simulink model "UUV_ss_reg"  (Simulink 8.0)
settings: Solver=ode45  StartTime=0.0  StopTime=10  RelTol=1e-3
values from neighbouring files (symbols this model uses):
  P =     [matlab.mat]
undefined symbols (not defined in the file or in its folder): controller, drawUUV
settings Model: Creator=beard  LastModifiedBy=tmclain
settings DataIOCC: SignalLoggingSaveFormat=ModelDataLogs
settings OptimizationCC: InitFltsAndDblsToZero=on
settings DebuggingCC: FcnCallInpInsideContextMsg=EnableAllAsWarning  StrictBusMsg=Warning
settings GRTTargetCC: CombineOutputUpdateFcns=off  GRTInterface=on

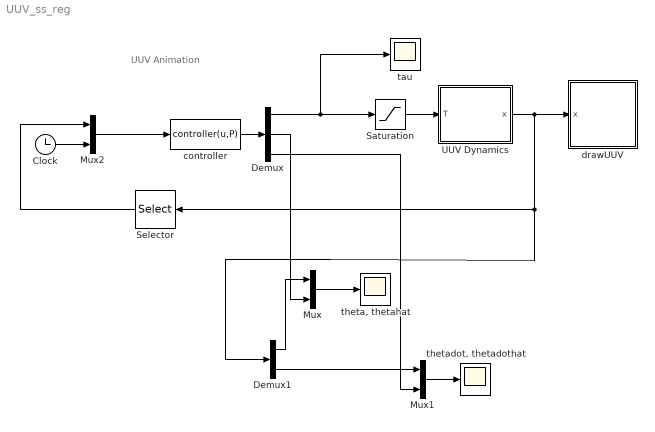
== system UUV_ss_reg ==
  note: UUV Animation
  Clock : Clock
  Demux : Demux  Outputs=3
  Demux1 : Demux  Outputs=2
  Mux : Mux  Inputs=2
  Mux1 : Mux  Inputs=2
  Mux2 : Mux  Inputs=2
  Saturation : Saturate  UpperLimit=250  LowerLimit=-250
  Selector : Selector  InputPortWidth=2  IndexOptions=Index vector (dialog)  Indices=[1]  OutputSizes=1
  UUV Dynamics : Subsystem
  controller : MATLABFcn  MATLABFcn=controller(u,P)  OutputDimensions=3  SampleTime=P.Ts
  drawUUV : Subsystem
      mask init:
      | % drawing parameters
      | MajorAxis = 10;
      | MinorAxis = 6;
      | C_M = [0;-4];
      mask Display: image(imread('tv.jpg'))
  tau : Scope
      settings: TimeRange=10  YMin=-500  YMax=100
  "theta, thetahat" : Scope
      settings: TimeRange=10  YMin=-0.1  YMax=0.6000000000000001  SaveName=ScopeData2
  "thetadot, thetadothat" : Scope
      settings: TimeRange=10  YMin=-1  YMax=4
  wires:
  UUV Dynamics/1(x) -> drawUUV/1(x), Selector/1, Demux1/1
  Saturation/1 -> UUV Dynamics/1(T)
  controller/1 -> Demux/1
  Demux/1 -> Saturation/1, tau/1
  Mux/1 -> "theta, thetahat"/1
  Demux1/1 -> Mux/1
  Demux/2 -> Mux/2
  Demux1/2 -> Mux1/1
  Demux/3 -> Mux1/2
  Mux1/1 -> "thetadot, thetadothat"/1
  Mux2/1 -> controller/1
  Clock/1 -> Mux2/2
  Selector/1 -> Mux2/1

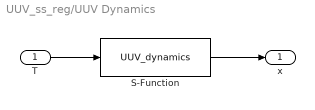
== system UUV_ss_reg/UUV Dynamics ==
  T : Inport
  S-Function : S-Function  FunctionName=UUV_dynamics  Parameters=P  EnableBusSupport=off
  x : Outport
  wires:
  T/1 -> S-Function/1
  S-Function/1 -> x/1

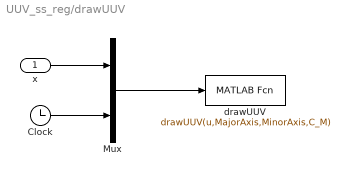
== system UUV_ss_reg/drawUUV ==
  x : Inport
  Clock : Clock
  Mux : Mux  Inputs=2
  drawUUV : MATLABFcn  MATLABFcn=drawUUV(u,MajorAxis,MinorAxis,C_M)  OutputDimensions=0  SampleTime=0.1
  wires:
  Mux/1 -> drawUUV/1
  x/1 -> Mux/1
  Clock/1 -> Mux/2
